simulink library "twolinkslib"  (R2016a)
settings: Solver=VariableStepAuto  StartTime=0.0  StopTime=10.0  RelTol=1e-3
settings Model: Creator=hqi  LastModifiedBy=hqi
settings GRTTargetCC: GeneratePreprocessorConditionals=Use local settings

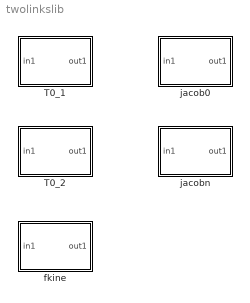
== system twolinkslib ==
  T0_1 : MATLAB Function  TreatAsAtomicUnit=on
  T0_2 : MATLAB Function  TreatAsAtomicUnit=on
  fkine : MATLAB Function  TreatAsAtomicUnit=on
  jacob0 : MATLAB Function  TreatAsAtomicUnit=on
  jacobn : MATLAB Function  TreatAsAtomicUnit=on

== matlab function twolinkslib/T0_1 ==
  data: in1 input; out1 output
function out1 = T0_1(in1)
%#codegen

%    This function was generated by the Symbolic Math Toolbox version 7.0.
%    29-Aug-2018 15:36:02

q1 = in1(:,1);
t2 = cos(q1);
t3 = sin(q1);
t4 = t3.*6.123233995736766e-17;
out1 = reshape([t2,t4,t3,0.0,-t3,t2.*6.123233995736766e-17,t2,0.0,0.0,-1.0,6.123233995736766e-17,0.0,t2,t4,t3,1.0],[4,4]);

== matlab function twolinkslib/fkine ==
  data: in1 input; out1 output
function out1 = fkine(in1)
%#codegen

%    This function was generated by the Symbolic Math Toolbox version 7.0.
%    29-Aug-2018 15:36:01

q1 = in1(:,1);
q2 = in1(:,2);
t2 = q1+q2;
t3 = cos(t2);
t4 = sin(t2);
t5 = t4.*6.123233995736766e-17;
t6 = sin(q1);
out1 = reshape([t3,t5,t4,0.0,-t4,t3.*6.123233995736766e-17,t3,0.0,0.0,-1.0,6.123233995736766e-17,0.0,t3+cos(q1),t5+t6.*6.123233995736766e-17,t4+t6,1.0],[4,4]);

== matlab function twolinkslib/T0_2 ==
  data: in1 input; out1 output
function out1 = T0_2(in1)
%#codegen

%    This function was generated by the Symbolic Math Toolbox version 7.0.
%    29-Aug-2018 15:36:02

q1 = in1(:,1);
q2 = in1(:,2);
t2 = cos(q1);
t3 = sin(q2);
t4 = cos(q2);
t5 = sin(q1);
t6 = t2.*t4;
t7 = t2.*t3.*6.123233995736766e-17;
t8 = t4.*t5.*6.123233995736766e-17;
t9 = t6-t3.*t5;
t10 = t2.*t3;
t11 = t4.*t5;
out1 = reshape([t9,t7+t8,t10+t11,0.0,-t2.*t3-t4.*t5,t2.*t4.*6.123233995736766e-17-t3.*t5.*6.123233995736766e-17,t9,0.0,0.0,-1.0,6.123233995736766e-17,0.0,t2+t6-t3.*t5,t5.*6.123233995736766e-17+t7+t8,t5+t10+t11,1.0],[4,4]);

== matlab function twolinkslib/jacob0 ==
  data: in1 input; out1 output
function out1 = jacob0(in1)
%#codegen

%    This function was generated by the Symbolic Math Toolbox version 7.0.
%    29-Aug-2018 15:36:07

q1 = in1(:,1);
q2 = in1(:,2);
t2 = q1+q2;
t3 = sin(t2);
t4 = cos(t2);
t5 = cos(q2);
t6 = t5+1.0;
t7 = sin(q2);
out1 = reshape([-t3.*t6+t4.*t7,t3.*t7.*6.123233995736766e-17+t4.*t6.*6.123233995736766e-17,t3.*t7+t4.*t6,0.0,-1.0,6.123233995736766e-17,-t3,t4.*6.123233995736766e-17,t4,0.0,-1.0,6.123233995736766e-17],[6,2]);

== matlab function twolinkslib/jacobn ==
  data: in1 input; out1 output
function out1 = jacobn(in1)
%#codegen

%    This function was generated by the Symbolic Math Toolbox version 7.0.
%    29-Aug-2018 15:36:07

q2 = in1(:,2);
out1 = reshape([sin(q2),cos(q2)+1.0,0.0,0.0,0.0,1.0,0.0,1.0,0.0,0.0,0.0,1.0],[6,2]);
